simulink model "cart"  (R2022a)
settings: Solver=VariableStepAuto  StartTime=0.0  StopTime=10.0  RelTol=1e-3
settings Model: Creator=Home  LastModifiedBy=Home

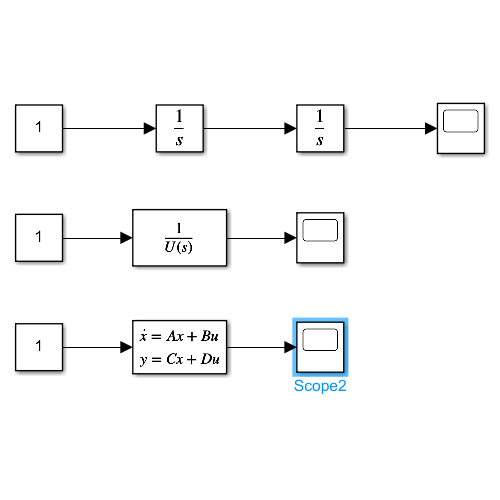
[thumbnail: Simulink's stored preview of the top-level diagram]
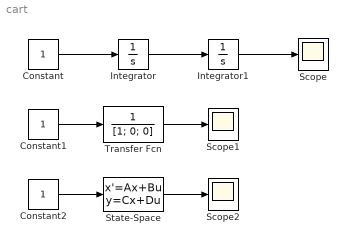
== system cart ==
  Constant : Constant
  Constant1 : Constant
  Constant2 : Constant
  Integrator : Integrator
  Integrator1 : Integrator
  Scope : Scope
  Scope1 : Scope
  Scope2 : Scope
  State-Space : StateSpace  A=[0 1; 0 0]  B=[0; 1]  C=[1 0]  InitialCondition=0
  Transfer Fcn : TransferFcn  Denominator=[1; 0; 0]
  wires:
  Integrator/1 -> Integrator1/1
  Integrator1/1 -> Scope/1
  Constant/1 -> Integrator/1
  Constant1/1 -> Transfer Fcn/1
  Transfer Fcn/1 -> Scope1/1
  Constant2/1 -> State-Space/1
  State-Space/1 -> Scope2/1
